simulink model "Lab9_Ideal_PID"  (R2016b)
settings: Solver=ode5  StartTime=0.0  StopTime=sim_stop_time  FixedStep=sim_step_size  RelTol=1e-3  EnableMultiTasking=on
values from neighbouring files (symbols this model uses):
  Bm = 0.0006001689451    [Lab9.mat]    (also in Lab9_JustinGarcia.m; lab9full.mat)
  Jm = 0.001321184025    [Lab9.mat]    (also in Lab9_JustinGarcia.m; lab9full.mat)
  Kb = 0.4952900056    [Lab9.mat]    (also in Lab9_JustinGarcia.m; lab9full.mat)
  Kd = 0    [Lab9.mat]    (also in Lab9_JustinGarcia.m; lab9full.mat)
  Ki = 38    [Lab9.mat]    (also in Lab9_JustinGarcia.m; lab9full.mat)
  Kp = 0.9    [Lab9.mat]    (also in Lab9_JustinGarcia.m; lab9full.mat)
  Kt = 0.3233728703    [Lab9.mat]    (also in Lab9_JustinGarcia.m; lab9full.mat)
  Lm = 0.0047    [Lab9.mat]    (also in Lab9_JustinGarcia.m; lab9full.mat)
  ref = [360 360 360 360 360 360 360 360 360 360 360 360 ... (124 elements, 124x1)]    [Lab9.mat]    (also in Lab9_JustinGarcia.m = 12; lab9full.mat)
  Rm = 5.262773292    [Lab9.mat]    (also in Lab9_JustinGarcia.m; lab9full.mat)
libraries: simulink x1
settings Model: Creator=009768408  LastModifiedBy=Mac
settings DataIOCC: LimitDataPoints=on  SaveFormat=Array
settings OptimizationCC: LifeSpan=inf
settings DebuggingCC: SFUnexpectedBacktrackingDiag=warning  SFNoUnconditionalDefaultTransitionDiag=warning  SFExecutionAtInitializationDiag=none
settings HardwareCC: ProdBitPerPointer=32  ProdBitPerSizeT=32  ProdBitPerPtrDiffT=32  ProdLargestAtomicFloat=None  ProdIntDivRoundTo=Undefined  ProdEndianess=Unspecified  ProdWordSize=32  ProdHWDeviceType=32-bit Generic
settings ModelReferenceCC: PropagateSignalLabelsOutOfModel=off
settings GRTTargetCC: TargetLangStandard=C89/C90 (ANSI)  GeneratePreprocessorConditionals=Disable all
settings ConfigComp: CovMetricSettings=dw  CovHtmlReporting=on  CovSaveCumulativeToWorkspaceVar=on  CovSaveSingleToWorkspaceVar=on  CovExternalEMLEnable=off

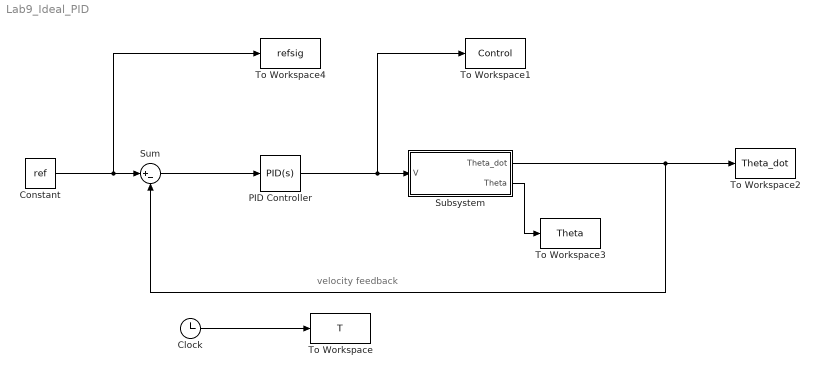
== system Lab9_Ideal_PID ==
  note: velocity feedback
  Clock : Clock
  Constant : Constant  Value=ref
  PID Controller : simulink/Continuous/PID Controller  Controller=PID  TimeDomain=Continuous-time  SampleTime=-1  IntegratorMethod=Forward Euler  FilterMethod=Forward Euler  Form=Parallel  UseFilter=on  ControllerParametersSource=internal  P=Kp  I=Ki  D=Kd  N=100  InitialConditionSource=internal  InitialConditionForIntegrator=0  InitialConditionForFilter=0  ExternalReset=none  LimitOutput=off  UpperSaturationLimit=inf  LowerSaturationLimit=-inf  LinearizeAsGain=on  AntiWindupMode=none  Kb=1  TrackingMode=off  Kt=1  PParamMin=[]  PParamMax=[]  IParamMin=[]  IParamMax=[]  DParamMin=[]  DParamMax=[]  NParamMin=[]  NParamMax=[]  KbParamMin=[]  KbParamMax=[]  KtParamMin=[]  KtParamMax=[]  POutMin=[]  POutMax=[]  IOutMin=[]  IOutMax=[]  DOutMin=[]  DOutMax=[]  NOutMin=[]  NOutMax=[]  KbOutMin=[]  KbOutMax=[]  KtOutMin=[]  KtOutMax=[]  IntegratorOutMin=[]  IntegratorOutMax=[]  FilterOutMin=[]  FilterOutMax=[]  SumOutMin=[]  SumOutMax=[]  SumI1OutMin=[]  SumI1OutMax=[]  SumI2OutMin=[]  SumI2OutMax=[]  SumI3OutMin=[]  SumI3OutMax=[]  SumDOutMin=[]  SumDOutMax=[]  SaturationOutMin=[]  SaturationOutMax=[]  IntegratorContinuousStateAttributes=''  IntegratorStateMustResolveToSignalObject=off  IntegratorRTWStateStorageClass=Auto  FilterContinuousStateAttributes=''  FilterStateMustResolveToSignalObject=off  FilterRTWStateStorageClass=Auto  DifferentiatorICPrevScaledInput=0  DifferentiatorOutMin=[]  DifferentiatorOutMax=[]
  Subsystem : Subsystem
  Sum : Sum  Inputs=|+-
  To Workspace : ToWorkspace  VariableName=T  SampleTime=-1
  To Workspace1 : ToWorkspace  VariableName=Control  SampleTime=-1
  To Workspace2 : ToWorkspace  VariableName=Theta_dot  SampleTime=-1
  To Workspace3 : ToWorkspace  VariableName=Theta  SampleTime=-1
  To Workspace4 : ToWorkspace  VariableName=refsig  SampleTime=-1
  wires:
  Clock/1 -> To Workspace/1
  Subsystem/2(Theta) -> To Workspace3/1
  PID Controller/1 -> To Workspace1/1, Subsystem/1(V)
  Sum/1 -> PID Controller/1
  Constant/1 -> To Workspace4/1, Sum/1
  Subsystem/1(Theta_dot) -> Sum/2, To Workspace2/1

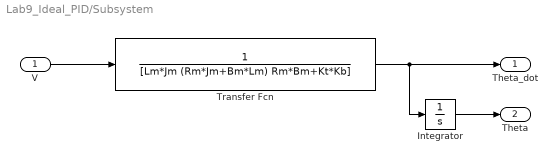
== system Lab9_Ideal_PID/Subsystem ==
  V : Inport
  Integrator : Integrator
  Transfer Fcn : TransferFcn  Denominator=[Lm*Jm (Rm*Jm+Bm*Lm) Rm*Bm+Kt*Kb]
  Theta_dot : Outport
  Theta : Outport  Port=2
  wires:
  Integrator/1 -> Theta/1
  Transfer Fcn/1 -> Integrator/1, Theta_dot/1
  V/1 -> Transfer Fcn/1
